simulink model "SIMULINK_03_INVERSE_CONTROL"  (R2020a)
settings: Solver=FixedStepAuto  StartTime=0.0  StopTime=500  FixedStep=0.001  RelTol=1e-3
libraries: simulink x1
settings Model: Creator=USUARIO  LastModifiedBy=USUARIO

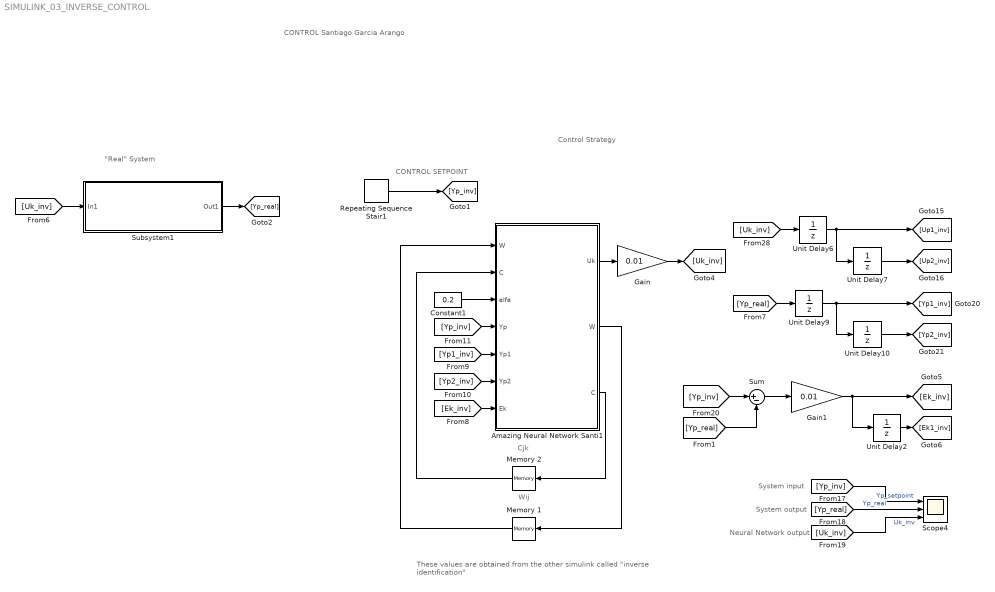
== system SIMULINK_03_INVERSE_CONTROL ==
  note: Control Strategy
  note: CONTROL SETPOINT
  note: System output
  note: System input
  note: Neural Network output
  note: "Real" System
  note: CONTROL
      | Santiago Garcia Arango
  note: Cjk
  note: Wij
  note: These values are obtained from the other simulink called
      | "inverse identification"
  " Memory 1" : Memory  InitialCondition=[-1.28120000000000,-0.553800000000000,-0.432200000000000;-0.185000000000000,-0.148800000000000,0.0194000000000000;-0.165100000000000,0.386600000000000,-2.91680000000000;1.52840000000000,-0.262700000000000,-0.458500000000000;-0.247700000000000,0.444700000000000,1.24360000000000;-1.10700000000000,0.348000000000000,-1.11180000000000;1.60310000000000,-1.25130000000000,0.932900000000000;1.22050000000000,-0.961700000000000,0.337100000000000;-0.237500000000000,-0.747800000000000,-0.0345000000000000;-1.52910000000000,-0.531200000000000,0.158600000000000]
  Amazing Neural Network Santi1 : MATLAB Function  TreatAsAtomicUnit=on
  Constant1 : Constant  Value=0.2
  Gain : Gain  Gain=0.01
  Gain1 : Gain  Gain=0.01
  Memory 2 : Memory  InitialCondition=[-1.52110000000000,-0.0418000000000000,1.58860000000000,0.0121000000000000,-0.0359000000000000,-0.672200000000000,-0.116900000000000,0.159900000000000,0.513400000000000,-0.311800000000000]
  Repeating Sequence Stair1 : simulink/Sources/Repeating Sequence Stair  OutValues=[0 0.2 0.1 0.3 0.4 0.3 0.2].'  tsamp=25  OutMin=[]  OutMax=[]  OutDataTypeStr=double  OutputDataTypeScalingMode=double  OutDataType=fixdt(0,8)  ConRadixGroup=Best Precision: Vector-wise  OutScaling=2^-12
  Scope4 : Scope  NumInputPorts=3
  Subsystem1 : Subsystem
  Sum : Sum  Inputs=|+-
  Unit Delay{2,6..7,9..10} (5 alike) : UnitDelay  SampleTime=-1  HasFrameUpgradeWarning=on
  wires:
  Repeating Sequence Stair1/1 -> [Yp_inv]
  [Yp_real] -> Sum/2
  [Yp_real] -> Scope4/2  "Yp_real"
  Sum/1 -> Gain1/1
  Unit Delay2/1 -> [Ek1_inv]
  Unit Delay7/1 -> [Up2_inv]
  [Yp_inv] -> Scope4/1  "Yp_setpoint"
  Unit Delay10/1 -> [Yp2_inv]
  [Uk_inv] -> Scope4/3  "Uk_inv"
  [Yp_real] -> Unit Delay9/1
  [Uk_inv] -> Unit Delay6/1
  Unit Delay9/1 -> [Yp1_inv], Unit Delay10/1
  Unit Delay6/1 -> [Up1_inv], Unit Delay7/1
  [Yp_inv] -> Sum/1
  Subsystem1/1(Out1) -> [Yp_real]
  [Uk_inv] -> Subsystem1/1(In1)
  Amazing Neural Network Santi1/3(C) -> Memory 2/1
  Constant1/1 -> Amazing Neural Network Santi1/3(alfa)
  Amazing Neural Network Santi1/2(W) -> " Memory 1"/1
  Memory 2/1 -> Amazing Neural Network Santi1/2("C ")
  [Ek_inv] -> Amazing Neural Network Santi1/7(Ek)
  [Yp1_inv] -> Amazing Neural Network Santi1/5(Yp1)
  " Memory 1"/1 -> Amazing Neural Network Santi1/1("W ")
  [Yp_inv] -> Amazing Neural Network Santi1/4(Yp)
  [Yp2_inv] -> Amazing Neural Network Santi1/6(Yp2)
  Amazing Neural Network Santi1/1(Uk) -> Gain/1
  Gain/1 -> [Uk_inv]
  Gain1/1 -> Unit Delay2/1, [Ek_inv]

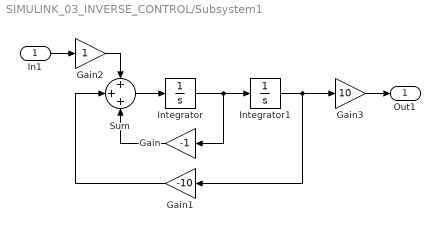
== system SIMULINK_03_INVERSE_CONTROL/Subsystem1 ==
  In1 : Inport
  Gain : Gain  Gain=-1
  Gain1 : Gain  Gain=-10
  Gain2 : Gain
  Gain3 : Gain  Gain=10
  Integrator : Integrator
  Integrator1 : Integrator
  Sum : Sum  Inputs=+++
  Out1 : Outport  VectorParamsAs1DForOutWhenUnconnected=off
  wires:
  Integrator/1 -> Integrator1/1, Gain/1
  Gain2/1 -> Sum/1
  Gain1/1 -> Sum/2
  Sum/1 -> Integrator/1
  Integrator1/1 -> Gain3/1, Gain1/1
  Gain/1 -> Sum/3
  In1/1 -> Gain2/1
  Gain3/1 -> Out1/1

== matlab function SIMULINK_03_INVERSE_CONTROL/Amazing Neural Network Santi1 ==
  data: W input; Uk output; C input; alfa input; Yp input; Yp1 input; Yp2 input; W output; C output; Ek input
% NEURAL NETWORK FOR SIMULINK "REAL-TIME" PROCESSING BASED ON SIGNALS
% Santiago Garcia Arango
% ------------------------------------------------------------------------
% FEEDFORWARDMADALINE. Train or Test a simple neural network.
%   alfa: Learning rate constant (1 x 1)
%   W: vector of the initial Weights. size (1 x ne)
%   C: matrix of the initial hidden layers weights. size (ns x no+1)
%   REMARK: This processing is based on an "Inverse Identification"
% ------------------------------------------------------------------------

function [Uk, W, C] = fcn(W, C, alfa, Yp, Yp1, Yp2, Ek)

activation_function_1 = "tanh";
activation_function_2 = "none";

X = [Yp Yp1 Yp2]; % Create "entries" vector
Aj = W*X'; % Add hidden layer

if (activation_function_1 == "tanh")
    H = tanh(Aj);
end

Ak = C'*H; % Add output layer

if (activation_function_2 == "none")
    Uk = Ak;
end

C = C+alfa*Ek*H; % Update weights of C

if (activation_function_1 == "tanh")
    H2 = sech(H).^2;
end

W = W+alfa*Ek*(C.*H2)*X; % Update weights of W

end
